simulink model "q1"  (R2020b)
settings: Solver=VariableStepAuto  StartTime=0.0  StopTime=10.0  RelTol=1e-3
undefined symbols (not defined in the file): k12, m2
settings Model: Creator=AVM  LastModifiedBy=AVM

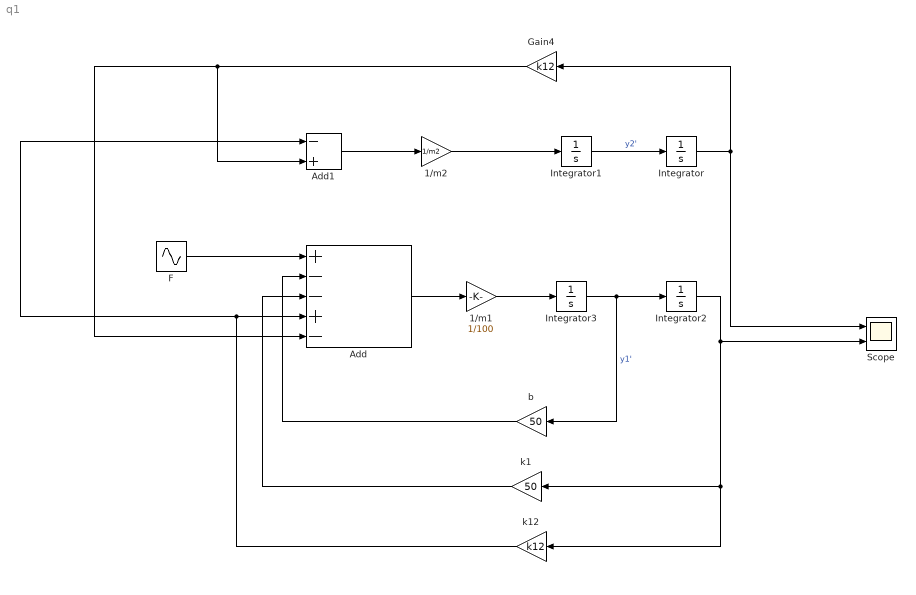
== system q1 ==
  1/m1 : Gain  Gain=1/100
  1/m2 : Gain  Gain=1/m2
  Add : Sum  Inputs=+--+-
  Add1 : Sum  Inputs=-+
  F : Sin  Amplitude=2  Frequency=10  SampleTime=0
  Gain4 : Gain  Gain=k12
  Integrator{,1..3} (4 alike) : Integrator
  Scope : Scope  NumInputPorts=2
  b : Gain  Gain=50
  k1 : Gain  Gain=50
  k12 : Gain  Gain=k12
  wires:
  k12/1 -> Add1/1, Add/4
  Add1/1 -> 1/m2/1
  Integrator/1 -> Scope/1, Gain4/1
  Gain4/1 -> Add1/2, Add/5
  1/m2/1 -> Integrator1/1
  k1/1 -> Add/3
  Add/1 -> 1/m1/1
  Integrator3/1 -> b/1, Integrator2/1  "y1'"
  1/m1/1 -> Integrator3/1
  b/1 -> Add/2
  F/1 -> Add/1
  Integrator2/1 -> Scope/2, k12/1, k1/1
  Integrator1/1 -> Integrator/1  "y2'"
